simulink model "LADRC_24a"  (R2024a)
settings: Solver=VariableStepAuto  StartTime=0  StopTime=10  FixedStep=0.001  RelTol=1e-5
model workspace (MAT data in the model file):
  Amp = 0.0011
  P = 0
values from neighbouring files (symbols this model uses):
  a = (1/Ms)*(bs+((Ke^2)/Rs))    (= 370.38637037)    [InitialParameter.m]
  b = 1    [InitialParameter.m]    (also in pneumatic_code.m = 0.0025)
  k1 = wc^4    (= 81450625)    [InitialParameter.m]    (also in pneumatic_code.m = 3620506.28125)
  k2 = 4*wc^3    (= 3429500)    [InitialParameter.m]    (also in pneumatic_code.m = 883050.3125)
  nh = 4    [InitialParameter.m]    (also in pneumatic_code.m)
  Pw = 0.0024    [InitialParameter.m]    (also in pneumatic_code.m = 0.0025)
  Ref = 0.001    [InitialParameter.m]
  Rh = 0.0019    [InitialParameter.m]    (also in pneumatic_code.m)
undefined symbols (not defined in the file or in its folder): L1, L2, L3
settings Model: Creator=ply  LastModifiedBy=pangl
settings OptimizationCC: ZeroExternalMemoryAtStartup=off  ZeroInternalMemoryAtStartup=off
settings DebuggingCC: UnderSpecifiedDimensionMsg=warning
settings RTWCC: TargetLang=C++
settings GRTTargetCC: TargetLangStandard=C++11 (ISO)  CodeInterfacePackaging=C++ class

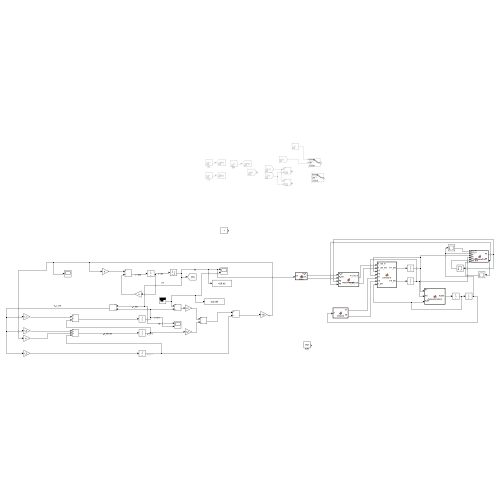
[thumbnail: Simulink's stored preview of the top-level diagram]
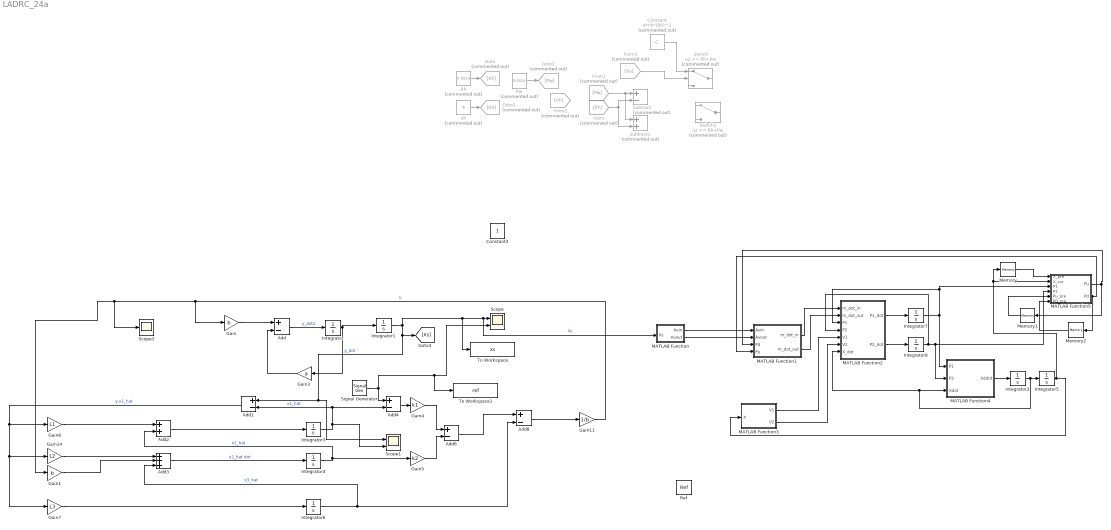
== system LADRC_24a ==
  Add{,1,4,6,8} (5 alike) : Sum  Inputs=+-
  Add2 : Sum
  Add3 : Sum  Inputs=+++
  Constant : Constant  Commented=on  Value=4*nh*(Rh)^2
  Constant3 : Constant
  From : From  Commented=on  GotoTag=Rh
  From1 : From  Commented=on  GotoTag=Pw
  From2 : From  Commented=on  GotoTag=nh
  From3 : From  Commented=on  GotoTag=Xs
  Gain : Gain  Gain=b
  Gain1 : Gain  Gain=b
  Gain11 : Gain  Gain=1/b
  Gain14 : Gain  Gain=L2
  Gain3 : Gain  Gain=a
  Gain4 : Gain  Gain=k1
  Gain5 : Gain  Gain=k2
  Gain6 : Gain  Gain=L1
  Gain7 : Gain  Gain=L3
  Goto : Goto  Commented=on  GotoTag=Rh
  Goto1 : Goto  Commented=on  GotoTag=nh
  Goto2 : Goto  Commented=on  GotoTag=Pw
  Integrator{,2..8} (8 alike) : Integrator
  Integrator1 : Integrator  LimitOutput=on  UpperSaturationLimit=0.0011  LowerSaturationLimit=-0.0011
  MATLAB Function : MATLAB Function  TreatAsAtomicUnit=on
  MATLAB Function1 : MATLAB Function  TreatAsAtomicUnit=on
  MATLAB Function2 : MATLAB Function  TreatAsAtomicUnit=on
  MATLAB Function3 : MATLAB Function  TreatAsAtomicUnit=on
  MATLAB Function4 : MATLAB Function  TreatAsAtomicUnit=on
  MATLAB Function5 : MATLAB Function  TreatAsAtomicUnit=on
  Memory : Memory
  Memory1 : Memory
  Memory2 : Memory
  Pw : Constant  Commented=on  Value=0.0024
  Ref : Constant  Value=Ref
  Rh : Constant  Commented=on  Value=0.0019
  Scope : Scope  NumInputPorts=2
  Scope1 : Scope  NumInputPorts=2
  Scope3 : Scope
  Signal Generator : SignalGenerator  WaveForm=square  Amplitude=0.0011
  Subtract : Sum  Commented=on  Inputs=+-
  Subtract1 : Sum  Commented=on
  Switch : Switch  Commented=on  Threshold=Rh+Pw  SaturateOnIntegerOverflow=off  InputSameDT=off
  Switch1 : Switch  Commented=on  Threshold=Rh+Pw  SaturateOnIntegerOverflow=off  InputSameDT=off
  To Workspace : ToWorkspace  VariableName=xs  SaveFormat=Structure  SampleTime=-1
  To Workspace1 : ToWorkspace  VariableName=ref  SaveFormat=Structure  SampleTime=-1
  nh : Constant  Commented=on  Value=4
  wires:
  Integrator/1 -> Integrator1/1, Gain3/1  "y_dot"
  Integrator1/1 -> [Xs], Add1/1, Scope1/1, To Workspace/1, MATLAB Function/1(Xs), Scope/1  "Xs"
  Add/1 -> Integrator/1  "y_dot2"
  Gain/1 -> Add/1
  Gain3/1 -> Add/2
  Integrator3/1 -> Scope1/2, Add1/2, Add4/2  "x1_hat"
  Add2/1 -> Integrator3/1
  Integrator4/1 -> Gain5/1, Add2/2  "x2_hat"
  Add3/1 -> Integrator4/1  "x2_hat dot"
  Gain14/1 -> Add3/1
  Add1/1 -> Gain14/1, Gain7/1, Gain6/1  "y-x1_hat"
  Gain7/1 -> Integrator6/1
  Gain11/1 -> Gain/1, Scope3/1, Gain1/1  "u"
  Gain6/1 -> Add2/1
  Add4/1 -> Gain4/1
  Gain1/1 -> Add3/2
  Gain4/1 -> Add6/1
  Gain5/1 -> Add6/2
  Add6/1 -> Add8/1
  Integrator6/1 -> Add3/3, Add8/2  "x3_hat"
  Add8/1 -> Gain11/1
  Signal Generator/1 -> Add4/1, To Workspace1/1, Scope/2
  MATLAB Function4/1(Xddot) -> Integrator2/1
  Integrator2/1 -> MATLAB Function2/7(X_dot), MATLAB Function4/3(Xdot), Integrator5/1
  MATLAB Function/1(Avin) -> MATLAB Function1/1(Avin)
  MATLAB Function/2(Avout) -> MATLAB Function1/2(Avout)
  MATLAB Function1/1(m_dot_in) -> MATLAB Function2/1(m_dot_in)
  MATLAB Function1/2(m_dot_out) -> MATLAB Function2/2(m_dot_out)
  MATLAB Function3/1(V1) -> MATLAB Function2/5(V1)
  MATLAB Function3/2(V2) -> MATLAB Function2/6(V2)
  Integrator5/1 -> Memory/1, MATLAB Function5/2(X_cur), MATLAB Function3/1(X)
  MATLAB Function2/1(P1_dot) -> Integrator7/1
  MATLAB Function2/2(P2_dot) -> Integrator8/1
  Integrator8/1 -> MATLAB Function2/4(P2), MATLAB Function5/4(P2), MATLAB Function4/2(P2)
  Integrator7/1 -> MATLAB Function2/3(P1), MATLAB Function5/3(P1), MATLAB Function4/1(P1)
  Memory/1 -> MATLAB Function5/1(X_pre)
  MATLAB Function5/1(Pu) -> MATLAB Function1/3(Pd), Memory1/1
  MATLAB Function5/2(Pd) -> Memory2/1, MATLAB Function1/4(Pu)
  Memory1/1 -> MATLAB Function5/5(Pu_pre)
  Memory2/1 -> MATLAB Function5/6(PD_pre)
  Rh/1 -> Goto/1
  nh/1 -> Goto1/1
  Pw/1 -> Goto2/1
  From1/1 -> Subtract1/1, Subtract/1
  From/1 -> Subtract1/2, Subtract/2
  From3/1 -> Switch/2
  Constant/1 -> Switch/1

== matlab function LADRC_24a/MATLAB Function1 ==
  data: Avin input; Avout input; m_dot_in output; Pd input; Pu input; m_dot_out output
function [m_dot_in,m_dot_out] = massflowrate(Avin,Avout,Pd,Pu)
% C1 = sqrt(k/R*(2/(k+1)^((k+1)/(k-1))));
% C2 = sqrt(2*k/(R*(k-1)));
%Pu = 758420;

C1 = 0.0404;
C2 = 0.1561;
Pcr = 0.528;
Cf=0.25;
k = 1.4;
T = 294;
if (Pd/Pu)<Pcr
    m_dot_in = Cf*Avin*C1*Pu/sqrt(T);
    m_dot_out = Cf*Avout*C1*Pu/sqrt(T);
elseif (Pd/Pu)>Pcr
    m_dot_in = Cf*Avin*C2*Pu/sqrt(T)*(Pd/Pu)^(1/k)*sqrt(1-((Pd/Pu)^((k-1)/k)));
    m_dot_out = Cf*Avout*C2*Pu/sqrt(T)*(Pd/Pu)^(1/k)*sqrt(1-((Pd/Pu)^((k-1)/k)));
else
    m_dot_in = 0;
    m_dot_out = 0;
end

    
end

== matlab function LADRC_24a/MATLAB Function ==
  data: Xs input; Avin output; Avout output
function [Avin,Avout]= area(Xs)
nh = 4;
Pw = 0.0024;
Rh = 0.0019;
sq = sqrt(abs((Rh-Pw+Xs)/(Rh+Pw-Xs)))
ph1 = 2*(Rh^2)*atan(sq)-((Pw-Xs)*sqrt(complex((Rh^2) - (Pw - Xs)^2)));
ph2 = 2*Rh^2*atan(sqrt((Rh-Pw+abs(Xs))/(Rh+Pw-abs(Xs))))-(Pw-abs(Xs))*sqrt(Rh^2 - (Pw - abs(Xs))^2);
%Avin=0;
%Avout=0;
if Xs<=Pw-Rh
    Avin = 0;
elseif (Pw-Rh<Xs)&&(Xs<Pw+Rh)
    Avin = nh*ph1;
else
    Avin = pi*nh*Rh^2;
end

if Xs<=-Pw-Rh
    Avout = pi*nh*Rh^2;
elseif (-Pw-Rh<Xs)&&(Xs<-Pw+Rh)
    Avout = nh*ph2;
else
    Avout = 0;
end

end

== matlab function LADRC_24a/MATLAB Function2 ==
  data: P1_dot output; m_dot_in input; m_dot_out input; P2_dot output; P1 input; P2 input; V1 input; V2 input; X_dot input
function [P1_dot,P2_dot] = pressure(m_dot_in, m_dot_out,P1,P2,V1,V2,X_dot)
A1 = 113.1e-6;
A2 = 95e-6;
R = 287;
T = 294;
k = 1.4;
a = 1.4;
P1_dot = R*T*k/V1*(a*m_dot_in-a*m_dot_out)-a*P1*A1/V1*X_dot;
P2_dot = R*T*k/V2*(a*m_dot_out-a*m_dot_in)-a*P2*A2/V2*X_dot;

end

== matlab function LADRC_24a/MATLAB Function3 ==
  data: V1 output; V2 output; X input
function [V1,V2] = Volume(X)
V01 = 10e-4;
V02 = 10e-4;
L = 0.15;
A1 = 113.1e-6;
A2 = 95e-6;
V1 = V01+(A1*X);
V2 = V02+(A2*(L-X));

end

== matlab function LADRC_24a/MATLAB Function4 ==
  data: P1 input; Xddot output; P2 input; Xdot input
function Xddot = dynamicmotion(P1,P2,Xdot)
Mpl = 0.1;
Pa = 101.35e3;
A1 = 113.1e-6;
A2 = 95e-6;
Ar = 50.26e-6;
b = 50;
Xddot = (P1*A1-P2*A2-Pa*Ar-b*Xdot)/(Mpl);

end

== matlab function LADRC_24a/MATLAB Function5 ==
  data: X_pre input; Pu output; Pd output; X_cur input; P1 input; P2 input; Pu_pre input; PD_pre input
function [Pu,Pd] = pressureFnc(X_pre,X_cur,P1,P2,Pu_pre,PD_pre)
Pa = 101.35e3;
Xd = X_cur - X_pre;

if(Xd>0)
    Pu = P1;
    Pd = P2;
elseif(Xd<0)
    Pu = P2;
    Pd = P1;
else
    Pu = Pu_pre;
    Pd = PD_pre;
end

end
